simulink model "A3_A8_Model_Final"  (R2023b)
settings: Solver=VariableStepAuto  StartTime=0.0  StopTime=10.0  RelTol=1e-3
settings Model: Creator=nikhi  LastModifiedBy=nikhi
settings DebuggingCC: ParameterPrecisionLossMsg=none

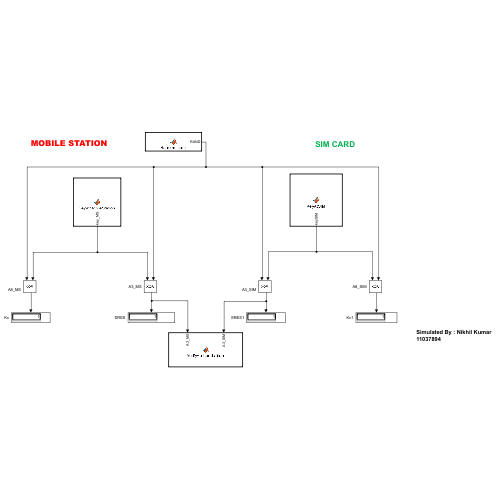
[thumbnail: Simulink's stored preview of the top-level diagram]
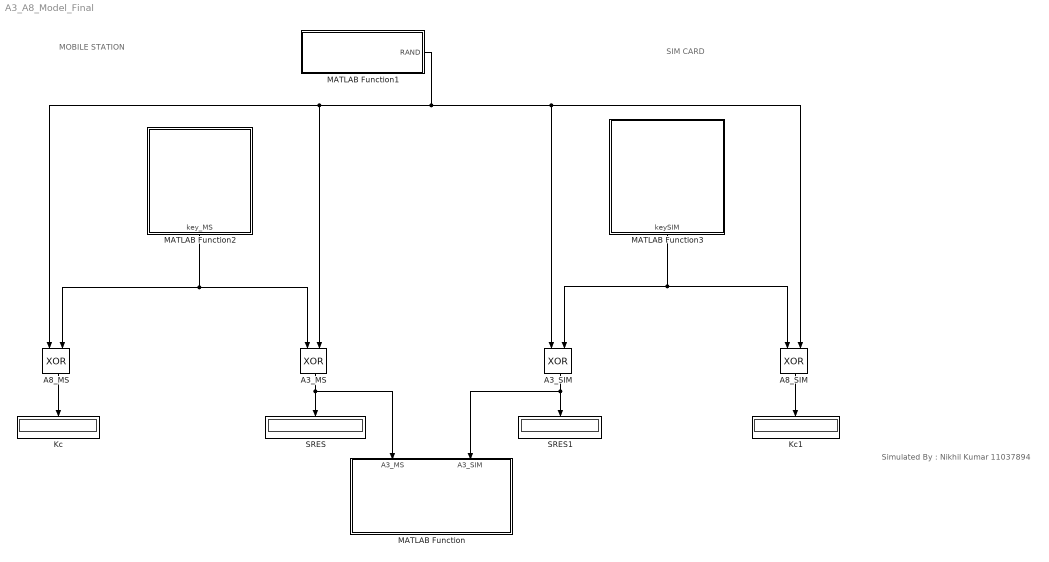
== system A3_A8_Model_Final ==
  note: Simulated By : Nikhil Kumar
      | 11037894
  note: SIM CARD
  note: MOBILE STATION
  " A3_SIM" : Logic  Operator=XOR  AllPortsSameDT=off  OutDataTypeStr=boolean
  " A8_MS" : Logic  Operator=XOR  AllPortsSameDT=off  OutDataTypeStr=boolean
  A3_MS : Logic  Operator=XOR  AllPortsSameDT=off  OutDataTypeStr=boolean
  A8_SIM : Logic  Operator=XOR  AllPortsSameDT=off  OutDataTypeStr=boolean
  Kc : Display
  Kc1 : Display
  MATLAB Function : MATLAB Function  TreatAsAtomicUnit=on
  MATLAB Function1 : MATLAB Function  TreatAsAtomicUnit=on
  MATLAB Function2 : MATLAB Function  TreatAsAtomicUnit=on
  MATLAB Function3 : MATLAB Function  TreatAsAtomicUnit=on
  SRES : Display
  SRES1 : Display
  wires:
  MATLAB Function1/1(RAND) -> " A3_SIM"/1, A8_SIM/2, A3_MS/2, " A8_MS"/1
  MATLAB Function2/1(key_MS) -> A3_MS/1, " A8_MS"/2
  A3_MS/1 -> MATLAB Function/1(A3_MS), SRES/1
  " A8_MS"/1 -> Kc/1
  MATLAB Function3/1(keySIM) -> " A3_SIM"/2, A8_SIM/1
  A8_SIM/1 -> Kc1/1
  " A3_SIM"/1 -> MATLAB Function/2(A3_SIM), SRES1/1

== matlab function A3_A8_Model_Final/MATLAB Function1 ==
  data: RAND output

function RAND = RandomInput()
    % Your custom MATLAB function logic here
    RAND = randi([0, 1], 1, 128);  % 128-bit random number
end

== matlab function A3_A8_Model_Final/MATLAB Function ==
  data: A3_MS input; A3_SIM input
function VerifyAuthentication(A3_MS, A3_SIM)
    % Verify if SRES1 equals SRES2  % Compare SRES1 and SRES2
    if (A3_MS==A3_SIM)
        disp('Authentication Successful');
    else
        disp('Authentication Not Successful');
    end
end

== matlab function A3_A8_Model_Final/MATLAB Function2 ==
  data: key_MS output
function key_MS = KeyAtMobileStation()
    % Your custom MATLAB function logic here
    key_MS = 111111111111111111111111111111111111111111111111111111111111111111111111111111111111111111111111111111111111111111111111111111111111111111111111111111111111111111111111111111111111111111111111111111111111111111111111111111111111111111;
end

== matlab function A3_A8_Model_Final/MATLAB Function3 ==
  data: keySIM output
function keySIM = KeyAtSIM()
    % Your custom MATLAB function logic here
    keySIM = 111111111111111111111111111111111111111111111111111111111111111111111111111111111111111111111111111111111111111111111111111111111111111111111111111111111111111111111111111111111111111111111111111111111111111111111111111111111111111111;
end
